simulink model "myDCMotorControl"  (R2019a)
settings: Solver=VariableStepAuto  StartTime=0.0  StopTime=10.0  RelTol=1e-3
undefined symbols (not defined in the file): PWMcmdMono, speedMono, Ts
settings Model: Creator=sb0526  LastModifiedBy=sb0526

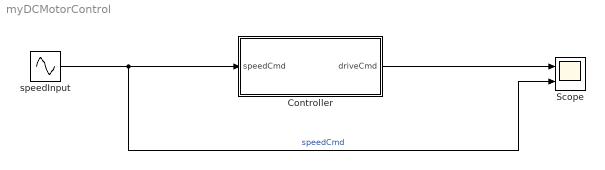
== system myDCMotorControl ==
  Controller : Subsystem
  Scope : Scope  NumInputPorts=2
  speedInput : Sin  Amplitude=6000  SampleTime=Ts
  wires:
  speedInput/1 -> Controller/1(speedCmd), Scope/2  "speedCmd"
  Controller/1(driveCmd) -> Scope/1

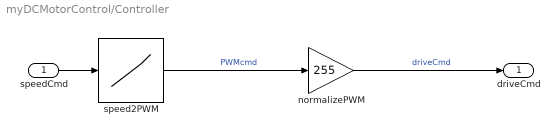
== system myDCMotorControl/Controller ==
  speedCmd : Inport
  normalizePWM : Gain  Gain=255
  "speed2PWM " : Lookup_n-D  NumberOfTableDimensions=1  BreakpointsForDimension1=speedMono  Table=PWMcmdMono  InternalRulePriority=Speed  RndMeth=Simplest  InputSameDT=on
  driveCmd : Outport
  wires:
  normalizePWM/1 -> driveCmd/1  "driveCmd"
  speedCmd/1 -> "speed2PWM "/1
  "speed2PWM "/1 -> normalizePWM/1  "PWMcmd"
